simulink model "Conventional_INC_MPPT"  (R2019b)
settings: Solver=ode23tb  StartTime=0.0  StopTime=4.5  RelTol=1e-3
libraries: powerlib x8, powerlib_meascontrol x2, re_lib x1
settings Model: SimulationMode=accelerator  Creator=FAST  LastModifiedBy=FAST

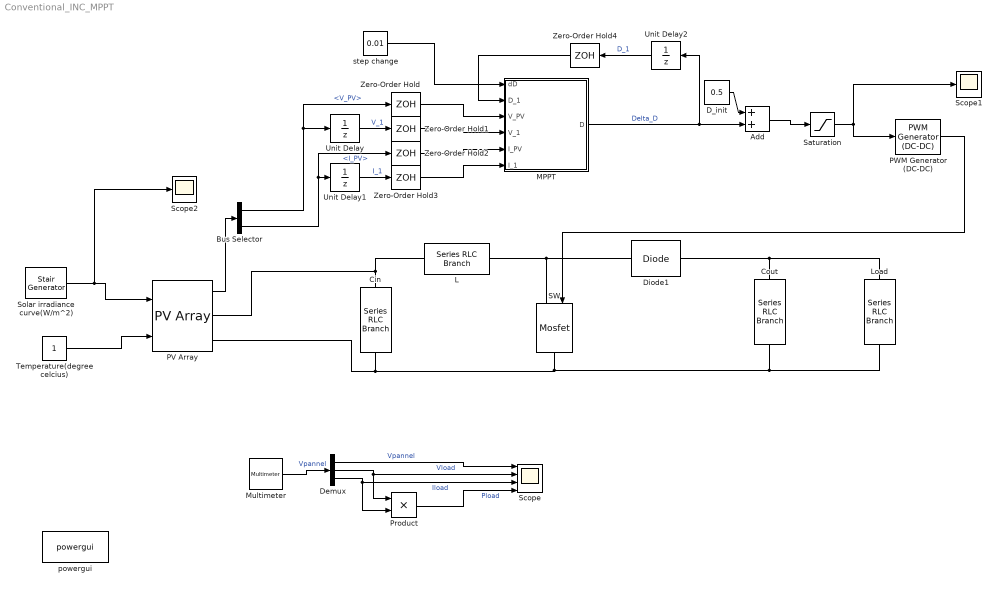
== system Conventional_INC_MPPT ==
  Add : Sum
  Bus Selector : BusSelector  OutputSignals=V_PV,I_PV
  Cin : powerlib/Elements/Series RLC Branch  LConnTagsString=__new0  RConnTagsString=__new0  BranchType=C  Resistance=1  Inductance=1e-3  SetiL0=off  InitialCurrent=0  Capacitance=470e-6  Setx0=off  InitialVoltage=0  Measurements=Branch voltage
      settings: SourceProductName=Simscape Electrical
  Cout : powerlib/Elements/Series RLC Branch  LConnTagsString=__new0  RConnTagsString=__new0  BranchType=C  Resistance=1  Inductance=1e-3  SetiL0=off  InitialCurrent=0  Capacitance=220e-6  Setx0=off  InitialVoltage=0  Measurements=None
      settings: SourceProductName=Simscape Electrical
  D_init : Constant  Value=0.5
  Demux : Demux  Outputs=3
  Diode1 : powerlib/Power Electronics/Diode  Ron=0.001  Lon=0  Vf=0.8  IC=0  UseSnubber=0  Rs=500  Cs=250e-9  Measurements=off
      settings: SourceProductName=Simscape Electrical
  L : powerlib/Elements/Series RLC Branch  LConnTagsString=__new0  RConnTagsString=__new0  BranchType=L  Resistance=1  Inductance=1e-3  SetiL0=off  InitialCurrent=0  Capacitance=200e-6  Setx0=off  InitialVoltage=0  Measurements=None
      settings: SourceProductName=Simscape Electrical
  Load : powerlib/Elements/Series RLC Branch  LConnTagsString=__new0  RConnTagsString=__new0  BranchType=R  Resistance=40  Inductance=1e-3  SetiL0=off  InitialCurrent=0  Capacitance=200e-6  Setx0=off  InitialVoltage=0  Measurements=Branch voltage and current
      settings: SourceProductName=Simscape Electrical
  MPPT : MATLAB Function  TreatAsAtomicUnit=on
  Multimeter : powerlib/Measurements/Multimeter  PhasorSimulation=off  OutputType=Complex  sel=[1 2 3]  L=3  Gain=[1 1 1]  yselected={'Ub: Cin','Ub: Load','Ib: Load'};  PSBOutputType=1  PSBequivalent=0  AxesSetting=[0,0.1,-100,100]  Display=0  SavedBlockNames=-11
      settings: SourceProductName=Simscape Electrical
  PV Array : re_lib/Solar/PV Array  Npar=1  Nser=1  PlotType=array @ 1000 W/m2 & specified temperatures  S_vec="[ 1000  500  100 ]"  Temp_C_vec="[ 45 25  ]"  ModuleName=STX Solar STX-245MT2  PlotWhenSelected=off  Pm=245.127  Ncell=60  Voc=38.02  Isc=8.82  Vm=30.3  Im=8.09  beta_Voc_pc=-0.3232  alpha_Isc_pc=0.038299  beta_Voc=-0.12288  alpha_Isc=0.003378  IL=8.8554  I0=7.421e-11  nI=0.96867  Rsh=100.7504  Rs=0.40489  BAL=on  Tc=1e-6  Tfilter=5e-5
      settings: SourceProductName=Simscape Electrical
  PWM Generator (DC-DC) : powerlib_meascontrol/Pulse & Signal Generators/PWM Generator (DC-DC)  Fsw=10000  Ts=0
      settings: SourceProductName=Simscape Electrical
  Product : Product
  SW : powerlib/Power Electronics/Mosfet  Ron=0.1  Lon=0  Rd=0.01  Vfd=0  IC=0  Rs=1e5  Cs=inf  Measurements=off
      settings: SourceProductName=Simscape Electrical
  Saturation : Saturate  UpperLimit=0.95  LowerLimit=0.01
  Scope : Scope  NumInputPorts=4
  Scope1 : Scope
  Scope2 : Scope
  Solar irradiance curve(W/m^2) : powerlib_meascontrol/Pulse & Signal Generators/Stair Generator  t=[0 0.8 2.8 4.5]  e="[400 900 400  400]"  Ts=0
      settings: SourceProductName=Simscape Electrical
  Temperature(degree celcius) : Constant
  Unit Delay : UnitDelay  SampleTime=0.05  HasFrameUpgradeWarning=on
  Unit Delay1 : UnitDelay  SampleTime=0.05  HasFrameUpgradeWarning=on
  Unit Delay2 : UnitDelay  SampleTime=0.05  HasFrameUpgradeWarning=on
  Zero-Order Hold{,1..3} (4 alike) : ZeroOrderHold  SampleTime=0.05
  Zero-Order Hold4 : ZeroOrderHold  SampleTime=0.05/60
  powergui : powerlib/powergui  Priority=1  SimulationMode=Continuous  SampleTime=1e-6  frequency=60  Iterations=50  frequencyindice=0  Pbase=100e6  ErrMax=1e-4  UnitsV=kV  UnitsW=MW  buscounter=0  FunctionMessages=off  echomessages=off  EnableUseOfTLC=off  CurrentSourceSwitches=off  DisableSnubberDevices=off  DisableRonSwitches=off  DisableVfSwitches=off  DisplayEquations=off  AutomaticDiscreteSolvers=off  SolverType=Tustin/Backward Euler (TBE)  Interpol=off  ExternalGateDelay=off  methode=off  Ts=100  x0status=blocks  SPID=on  SwTol=0  HookPort=off  NonlinearTolerance=1e-4  nMaxIteration=100  ContinueOnMaxIteration=off  RestoreLinks=warning  ResistiveCurrentMeasurement=off  Frange=[0:2:500]  Ylog=off  Xlog=on  ShowGrid=off  save=off  variable=ZData  structure=0  ZoomFFT=off  StartTime=0.0  cycles=1  DisplayStyle=1  fundamental=60  FreqAxis=off  MaxFrequency=1000  frequencyindicesteady=1  RmsSteady=1  display=off
      settings: SourceProductName=Simscape Electrical
  step change : Constant  Value=0.01
  wires:
  Solar irradiance curve(W/m^2)/1 -> Scope2/1, PV Array/1
  Temperature(degree celcius)/1 -> PV Array/2
  PV Array/1 -> Bus Selector/1
  Bus Selector/1 -> Zero-Order Hold/1, Unit Delay/1  "<V_PV>"
  Bus Selector/2 -> Zero-Order Hold2/1, Unit Delay1/1  "<I_PV>"
  Unit Delay/1 -> Zero-Order Hold1/1  "V_1"
  Unit Delay1/1 -> Zero-Order Hold3/1  "I_1"
  PWM Generator (DC-DC)/1 -> SW/1
  Zero-Order Hold/1 -> MPPT/3(V_PV)
  Zero-Order Hold1/1 -> MPPT/4(V_1)
  Zero-Order Hold2/1 -> MPPT/5(I_PV)
  Zero-Order Hold3/1 -> MPPT/6(I_1)
  MPPT/1(D) -> Unit Delay2/1, Add/2  "Delta_D"
  Saturation/1 -> PWM Generator (DC-DC)/1, Scope1/1
  Multimeter/1 -> Demux/1  "Vpannel"
  Demux/1 -> Scope/1  "Vpannel"
  Demux/2 -> Product/1, Scope/2  "Vload"
  Demux/3 -> Product/2, Scope/3  "Iload"
  Product/1 -> Scope/4  "Pload"
  step change/1 -> MPPT/1(dD)
  Unit Delay2/1 -> Zero-Order Hold4/1  "D_1"
  Zero-Order Hold4/1 -> MPPT/2(D_1)
  Add/1 -> Saturation/1
  D_init/1 -> Add/1
  connections:
  Cin/LConn1 -- L/LConn1 -- PV Array/RConn1
  Cin/RConn1 -- Load/RConn1 -- Cout/RConn1 -- SW/RConn1 -- PV Array/RConn2
  SW/LConn1 -- Diode1/LConn1 -- L/RConn1
  Diode1/RConn1 -- Load/LConn1 -- Cout/LConn1

== matlab function Conventional_INC_MPPT/MPPT ==
  data: dD input; D output; D_1 input; V_PV input; V_1 input; I_PV input; I_1 input
function D = fcn(dD,D_1,V_PV,V_1,I_PV,I_1)
dv=V_PV-V_1;
di=I_PV-I_1;
D=D_1;
if(dv==0)
    if(di~=0)
        if(di>0)
            D=D-dD;
        else
            D=D+dD;
        end
    end  
    
else
    if(di/dv~=-I_PV/V_PV)
       if(di/dv>-I_PV/V_PV)
            D=D-dD;
       else
            D=D+dD;
       end
        
    end
    
end
